simulink model "Practica_7_OPAMPs"  (R2022b)
settings: Solver=VariableStepAuto  StartTime=0.0  StopTime=10.0  RelTol=1e-3
values from neighbouring files (symbols this model uses):
  C1 = 100e-9    (= 1e-07)    [OPAMPs.m]    (also in Parametros_practica_7.m)
  C2 = 100e-9    (= 1e-07)    [OPAMPs.m]    (also in Parametros_practica_7.m)
  R1 = 5e6    (= 5000000)    [OPAMPs.m]    (also in Parametros_practica_7.m)
  R2 = 5e6    (= 5000000)    [OPAMPs.m]    (also in Parametros_practica_7.m)
  R3 = 5e6    (= 5000000)    [OPAMPs.m]    (also in Parametros_practica_7.m)
libraries: fl_lib x10, nesl_utility x2
settings Model: Creator=mluser  LastModifiedBy=josel
settings OptimizationCC: ReuseModelBlockBuffer=on

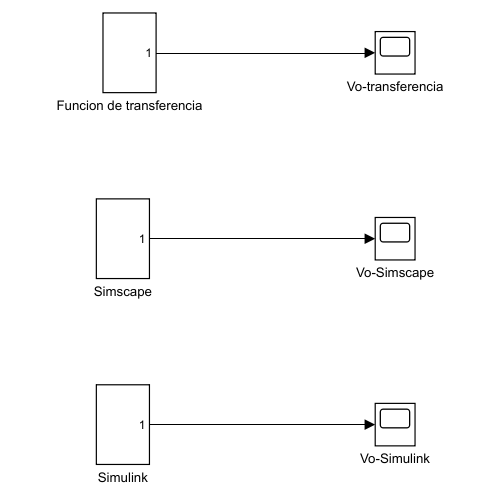
[thumbnail: Simulink's stored preview of the top-level diagram]
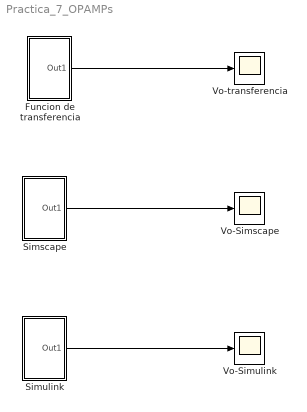
== system Practica_7_OPAMPs ==
  Funcion de transferencia : Subsystem
  Simscape : Subsystem
  Simulink : Subsystem
  Vo-Simscape : Scope
  Vo-Simulink : Scope
  Vo-transferencia : Scope
  wires:
  Simulink/1(Out1) -> Vo-Simulink/1
  Simscape/1(Out1) -> Vo-Simscape/1
  Funcion de transferencia/1(Out1) -> Vo-transferencia/1

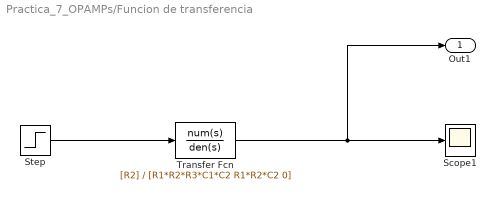
== system Practica_7_OPAMPs/Funcion de transferencia ==
  Scope1 : Scope
  Step : Step  Time=0  SampleTime=0
  Transfer Fcn : TransferFcn  Numerator=[R2]  Denominator=[R1*R2*R3*C1*C2 R1*R2*C2 0]
  Out1 : Outport
  wires:
  Step/1 -> Transfer Fcn/1
  Transfer Fcn/1 -> Out1/1, Scope1/1

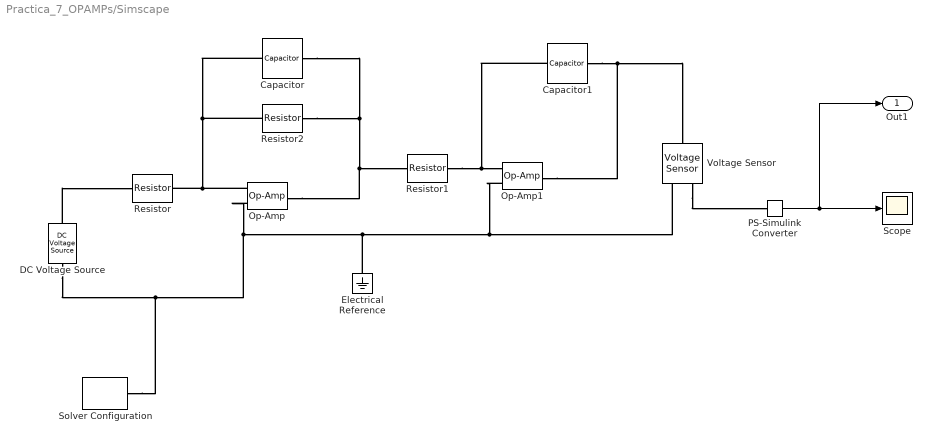
== system Practica_7_OPAMPs/Simscape ==
  Capacitor : fl_lib/Electrical/Electrical Elements/Capacitor  c=100 nF  r=1e-6 Ohm  g=0 1/Ohm  i_specify=off  i_priority=None  i=0 A  i_nominal_specify=off  i_nominal_unit=A  i_nominal_value=1  v_specify=off  v_priority=None  v=0 V  v_nominal_specify=off  v_nominal_unit=V  v_nominal_value=1  vc_specify=off  vc_priority=High  vc=0 V  vc_nominal_specify=off  vc_nominal_unit=V  vc_nominal_value=1
  Capacitor1 : fl_lib/Electrical/Electrical Elements/Capacitor  c=100 nF  r=1e-6 Ohm  g=0 1/Ohm  i_specify=off  i_priority=None  i=0 A  i_nominal_specify=off  i_nominal_unit=A  i_nominal_value=1  v_specify=off  v_priority=None  v=0 V  v_nominal_specify=off  v_nominal_unit=V  v_nominal_value=1  vc_specify=off  vc_priority=High  vc=0 V  vc_nominal_specify=off  vc_nominal_unit=V  vc_nominal_value=1
  DC Voltage Source : fl_lib/Electrical/Electrical Sources/DC Voltage Source  v0=1 V
  Electrical Reference : fl_lib/Electrical/Electrical Elements/Electrical Reference
  Op-Amp : fl_lib/Electrical/Electrical Elements/Op-Amp  outI_specify=off  outI_priority=None  outI=0 A  outI_nominal_specify=off  outI_nominal_unit=A  outI_nominal_value=1
  Op-Amp1 : fl_lib/Electrical/Electrical Elements/Op-Amp  outI_specify=off  outI_priority=None  outI=0 A  outI_nominal_specify=off  outI_nominal_unit=A  outI_nominal_value=1
  PS-Simulink Converter : nesl_utility/PS-Simulink Converter  PhysicalDomain=network_engine_domain  SubClassName=ps_output  LeftPortType=input  RightPortType=output  PseudoPeriodic=off  Frequencies=[]  VectorFormat=inherit  Unit=inherit  AffineConversion=off
  Resistor : fl_lib/Electrical/Electrical Elements/Resistor  R=5 MOhm  i_specify=off  i_priority=None  i=0 A  i_nominal_specify=off  i_nominal_unit=A  i_nominal_value=1  v_specify=off  v_priority=None  v=0 V  v_nominal_specify=off  v_nominal_unit=V  v_nominal_value=1
  Resistor1 : fl_lib/Electrical/Electrical Elements/Resistor  R=5 MOhm  i_specify=off  i_priority=None  i=0 A  i_nominal_specify=off  i_nominal_unit=A  i_nominal_value=1  v_specify=off  v_priority=None  v=0 V  v_nominal_specify=off  v_nominal_unit=V  v_nominal_value=1
  Resistor2 : fl_lib/Electrical/Electrical Elements/Resistor  R=5 MOhm  i_specify=off  i_priority=None  i=0 A  i_nominal_specify=off  i_nominal_unit=A  i_nominal_value=1  v_specify=off  v_priority=None  v=0 V  v_nominal_specify=off  v_nominal_unit=V  v_nominal_value=1
  Scope : Scope
  Solver Configuration : nesl_utility/Solver Configuration  PhysicalDomain=network_engine_domain  SubClassName=solver  LeftPortType=input  RightPortType=generic  Tones=[]  Harmonics=[]  SimulateNoise=off  Profile=off  UseLocalSampling=off  EnableSwitchedLinearOptims=on  FrequencyDomain=off  UseCCode=off  RelTol=0.001  AbsTol=0.001  MinStep=1e-09  ToWorkspace=off  RevertToSquareIcSolve=off  NumHomotopyIterations=100  PhasorMode=off  PhasorModeNumHarmonics=1  ConsistencySolver=NEWTON_XTOL_AFTER_FTOL  IndexReductionMethod=DerivativeReplacement  DoDC=off  ResidualTolerance=1e-09  ConsistencyTolSource=GLOBAL  ConsistencyAbsTol=0.001  ConsistencyRelTol=0.001  ConsistencyTolFactor=0.001  UseLocalSolver=off  LocalSolverChoice=NE_BACKWARD_EULER_ADVANCER  ResolveIndetEquations=on  FunctionEvalNumThread=1  LocalSolverSampleTime=0.001  DoFixedCost=off  MaxNonlinIter=3  MaxModeIter=2  ComputeImpulses=off  ImpulseIterations=2  LinearAlgebra=auto  LinearAlgebraNumThread=0  EquationFormulation=NE_TIME_EF  DelaysMemoryBudget=1024  AutomaticFiltering=on  FilteringTimeConstant=0.001  PartitionStorageMethod=AS_NEEDED  PartitionMemoryBudget=1024  PartitionMethod=ROBUST
  Voltage Sensor : fl_lib/Electrical/Electrical Sensors/Voltage Sensor
  Out1 : Outport
  wires:
  PS-Simulink Converter/1 -> Scope/1, Out1/1
  connections:
  Capacitor1/RConn1 -- Op-Amp1/RConn1 -- Voltage Sensor/LConn1
  Op-Amp/LConn2 -- Capacitor/LConn1 -- Resistor2/LConn1 -- Resistor/RConn1
  Op-Amp/LConn1 -- Solver Configuration/RConn1 -- DC Voltage Source/RConn1 -- Electrical Reference/LConn1 -- Op-Amp1/LConn1 -- Voltage Sensor/RConn2
  Op-Amp/RConn1 -- Capacitor/RConn1 -- Resistor2/RConn1 -- Resistor1/LConn1
  DC Voltage Source/LConn1 -- Resistor/LConn1
  Resistor1/RConn1 -- Capacitor1/LConn1 -- Op-Amp1/LConn2
  Voltage Sensor/RConn1 -- PS-Simulink Converter/LConn1

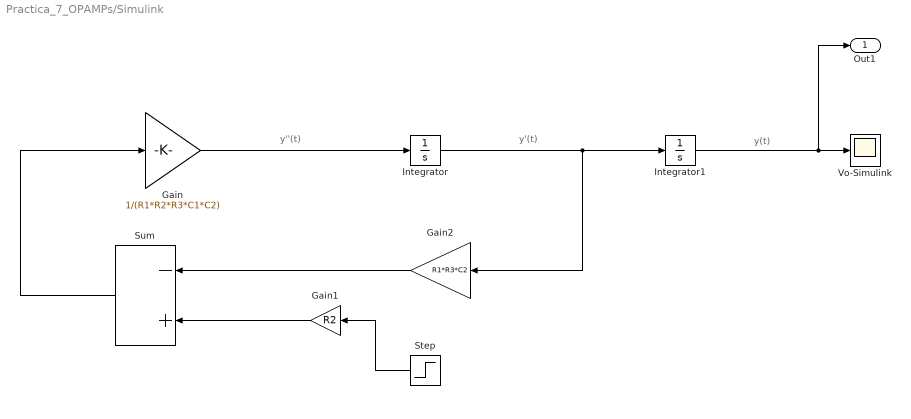
== system Practica_7_OPAMPs/Simulink ==
  note: y(t)
  note: y''(t)
  note: y'(t)
  Gain : Gain  Gain=1/(R1*R2*R3*C1*C2)
  Gain1 : Gain  Gain=R2
  Gain2 : Gain  Gain=R1*R3*C2
  Integrator : Integrator
  Integrator1 : Integrator
  Step : Step  Time=0  SampleTime=0
  Sum : Sum  Inputs=-+
  Vo-Simulink : Scope
  Out1 : Outport
  wires:
  Integrator/1 -> Gain2/1, Integrator1/1
  Gain2/1 -> Sum/1
  Gain/1 -> Integrator/1
  Step/1 -> Gain1/1
  Gain1/1 -> Sum/2
  Sum/1 -> Gain/1
  Integrator1/1 -> Out1/1, Vo-Simulink/1
